simulink library "csu_iqf_inertial_quat_feedback_lib"  (R2014b)
settings: Solver=ode45  StartTime=0.0  StopTime=10.0  RelTol=1e-3
libraries: util_quat_lib x4, util_common_lib x2, util_info_lib x1
settings Model: Creator=Nilesh  LastModifiedBy=mstewart

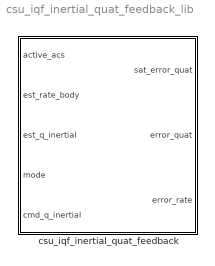
== system csu_iqf_inertial_quat_feedback_lib ==
  csu_iqf_inertial_quat_feedback : Subsystem

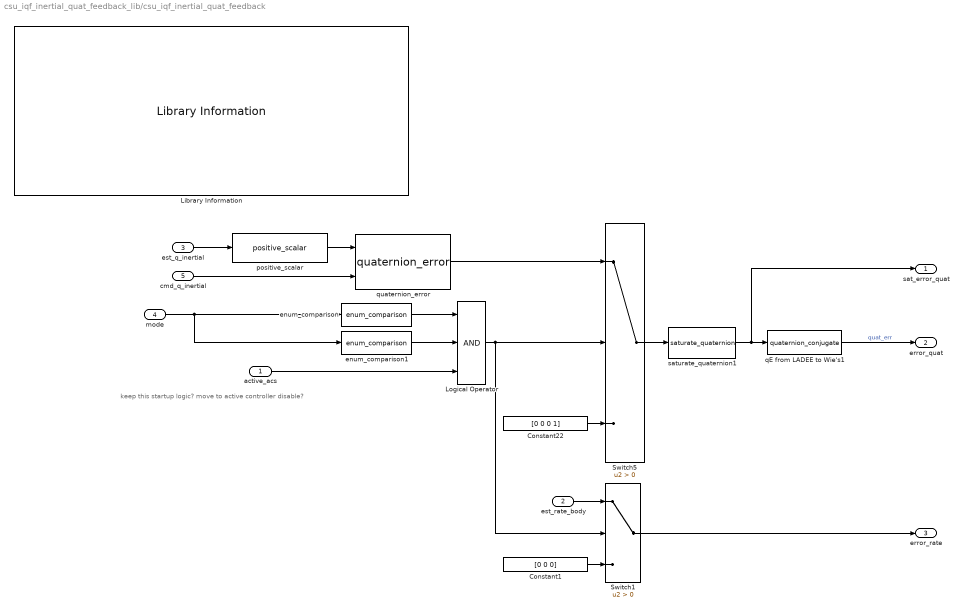
== system csu_iqf_inertial_quat_feedback_lib/csu_iqf_inertial_quat_feedback ==
  note: keep this startup logic? move to active controller disable?
  active_acs : Inport
  est_rate_body : Inport  Port=2
  est_q_inertial : Inport  Port=3
  mode : Inport  Port=4
  cmd_q_inertial : Inport  Port=5
  Constant1 : Constant  Value=[0 0 0]
  Constant22 : Constant  Value=[0 0 0 1]
  Library Information : util_info_lib/Library Information  owner='NONE'
  Logical Operator : Logic  Inputs=3  AllPortsSameDT=off  OutDataTypeStr=boolean
  Switch1 : Switch  Criteria=u2 > Threshold
  Switch5 : Switch  Criteria=u2 > Threshold
  enum_comparison : util_common_lib/enum_comparison  comparison_type=~=
  enum_comparison1 : util_common_lib/enum_comparison  comparison_type=~=
  positive_scalar : util_quat_lib/positive_scalar  SystemSampleTime=-1
  qE from LADEE to Wie's1 : util_quat_lib/quaternion_conjugate  SystemSampleTime=-1
  quaternion_error : util_quat_lib/quaternion_error  SystemSampleTime=-1
  saturate_quaternion1 : util_quat_lib/saturate_quaternion  theta_max=iqf_attitude_error_saturation_threshold
  sat_error_quat : Outport
  error_quat : Outport  Port=2
  error_rate : Outport  Port=3
  wires:
  Switch1/1 -> error_rate/1
  Constant1/1 -> Switch1/3
  est_rate_body/1 -> Switch1/1
  quaternion_error/1 -> Switch5/1
  saturate_quaternion1/1 -> qE from LADEE to Wie's1/1, sat_error_quat/1
  enum_comparison1/1 -> Logical Operator/2
  est_q_inertial/1 -> positive_scalar/1
  positive_scalar/1 -> quaternion_error/1
  cmd_q_inertial/1 -> quaternion_error/2
  qE from LADEE to Wie's1/1 -> error_quat/1  "quat_err"
  Switch5/1 -> saturate_quaternion1/1
  Constant22/1 -> Switch5/3
  Logical Operator/1 -> Switch5/2, Switch1/2
  enum_comparison/1 -> Logical Operator/1
  active_acs/1 -> Logical Operator/3
  mode/1 -> enum_comparison/1, enum_comparison1/1
